simulink model "airspeed_from_throttle_loop"  (R2016b)
settings: Solver=VariableStepAuto  StartTime=0.0  StopTime=10.0  RelTol=1e-3
undefined symbols (not defined in the file): a_V1, a_V2, k_i_v, k_p_v
settings Model: Creator=geun2  LastModifiedBy=geun2

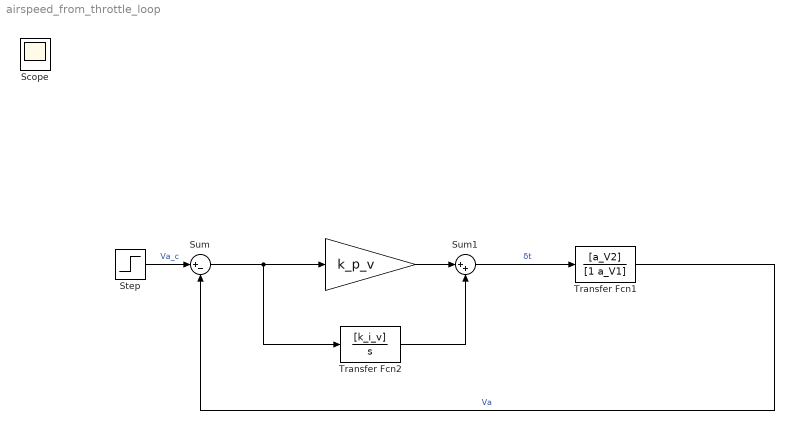
== system airspeed_from_throttle_loop ==
  " " : Gain  Gain=k_p_v
  Step : Step  SampleTime=0
  Sum : Sum  Inputs=|+-
  Sum1 : Sum  Inputs=|++
  Transfer Fcn1 : TransferFcn  Numerator=[a_V2]  Denominator=[1 a_V1]
  Transfer Fcn2 : TransferFcn  Numerator=[k_i_v]  Denominator=[1 0]
  Scope : Scope
  wires:
  Sum/1 -> Transfer Fcn2/1, " "/1
  Transfer Fcn1/1 -> Sum/2  "Va"
  Step/1 -> Sum/1  "Va_c"
  " "/1 -> Sum1/1
  Transfer Fcn2/1 -> Sum1/2
  Sum1/1 -> Transfer Fcn1/1  "δt"
